simulink model "Sim4_CTM_Uncertainty_Controller"  (R2019b)
settings: Solver=ode45  StartTime=0.0  StopTime=10  MaxStep=0.001  RelTol=1e-3
StopFcn:
  | Colors=hsv(5)';
  | for i=1:5
  | plot(out.tout,out.R_UCTM(:,i),'color',Colors(:,i),'LineWidth',1.5)
  | hold on
  | end
  | grid on
  | legend('Joint1','Joint2','Joint3','Joint4','Joint5')
  | title(['Response Vs Input of Joints Via UCTM'])
  | xlabel('Time')
  | ylabel('Response')
  | 
  | 
  | 
  | %plot(out.tout,out.Results,'LineWidth',1.3)
  | %grid on
  | %legend('Joint1','Joint2','Joint3','Joint4','Joint5')
  | %xlabel('Response')
  | %ylabel('Time')
libraries: simulink x5
(part 1 of 3)
settings Model: Creator=baran  LastModifiedBy=baran

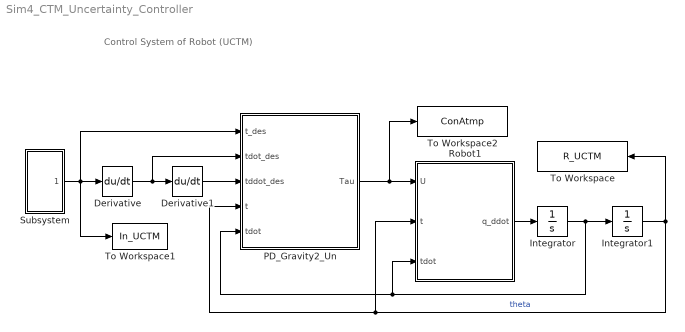
== system Sim4_CTM_Uncertainty_Controller ==
  note: Control System of Robot (UCTM)
  Derivative : Derivative
  Derivative1 : Derivative
  Integrator : Integrator  InitialCondition=[0 0 0 0 0]'
  Integrator1 : Integrator  InitialCondition=[-5 -4 -3 -2 -1]'
  PD_Gravity2_Un : MATLAB Function  TreatAsAtomicUnit=on
  Robot1 : MATLAB Function  TreatAsAtomicUnit=on
  Subsystem : Subsystem
  To Workspace : ToWorkspace  VariableName=R_UCTM  SampleTime=-1
  To Workspace1 : ToWorkspace  VariableName=In_UCTM  SampleTime=-1
  To Workspace2 : ToWorkspace  VariableName=ConAtmp  SampleTime=-1
  wires:
  PD_Gravity2_Un/1(Tau) -> To Workspace2/1, Robot1/1(U)
  Integrator/1 -> PD_Gravity2_Un/5(tdot), Robot1/3(tdot), Integrator1/1
  Robot1/1(q_ddot) -> Integrator/1
  Derivative/1 -> PD_Gravity2_Un/2(tdot_des), Derivative1/1
  Derivative1/1 -> PD_Gravity2_Un/3(tddot_des)
  Integrator1/1 -> PD_Gravity2_Un/4(t), Robot1/2(t), To Workspace/1  "theta"
  Subsystem/1(INPUT) -> PD_Gravity2_Un/1(t_des), To Workspace1/1, Derivative/1

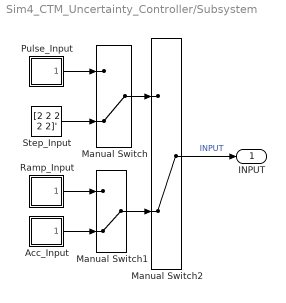
== system Sim4_CTM_Uncertainty_Controller/Subsystem ==
  Acc_Input : Subsystem
  Manual Switch : ManualSwitch  CurrentSetting=0
  Manual Switch1 : ManualSwitch  CurrentSetting=0
  Manual Switch2 : ManualSwitch  CurrentSetting=0
  Pulse_Input : Subsystem
  Ramp_Input : Subsystem
  Step_Input : Constant  Value=[2 2 2 2 2]'
  INPUT : Outport
  wires:
  Acc_Input/1(INPUT) -> Manual Switch1/2
  Ramp_Input/1(INPUT) -> Manual Switch1/1
  Pulse_Input/1(INPUT) -> Manual Switch/1
  Manual Switch2/1 -> INPUT/1  "INPUT"
  Manual Switch/1 -> Manual Switch2/1
  Manual Switch1/1 -> Manual Switch2/2
  Step_Input/1 -> Manual Switch/2

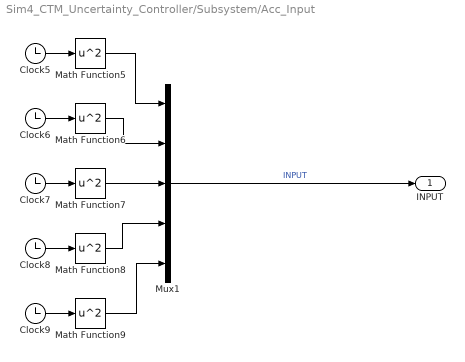
== system Sim4_CTM_Uncertainty_Controller/Subsystem/Acc_Input ==
  Clock{5..9} (5 alike) : Clock
  Math Function{5..9} (5 alike) : Math  Operator=square  SignedPower=off  SaturateOnIntegerOverflow=on
  Mux1 : Mux  Inputs=5
  INPUT : Outport
  wires:
  Math Function8/1 -> Mux1/4
  Math Function9/1 -> Mux1/5
  Clock5/1 -> Math Function5/1
  Math Function7/1 -> Mux1/3
  Clock9/1 -> Math Function9/1
  Math Function6/1 -> Mux1/2
  Clock8/1 -> Math Function8/1
  Clock7/1 -> Math Function7/1
  Math Function5/1 -> Mux1/1
  Clock6/1 -> Math Function6/1
  Mux1/1 -> INPUT/1  "INPUT"

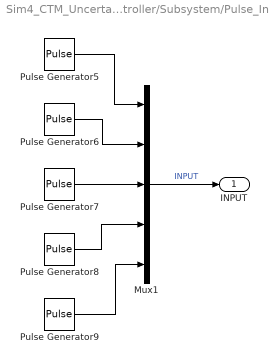
== system Sim4_CTM_Uncertainty_Controller/Subsystem/Pulse_Input ==
  Mux1 : Mux  Inputs=5
  Pulse Generator5 : DiscretePulseGenerator  PulseType=Time based  Period=10  PulseWidth=0.1
  Pulse Generator6 : DiscretePulseGenerator  PulseType=Time based  Amplitude=0.5  Period=10  PulseWidth=0.1
  Pulse Generator7 : DiscretePulseGenerator  PulseType=Time based  Amplitude=0.25  Period=10  PulseWidth=0.1
  Pulse Generator8 : DiscretePulseGenerator  PulseType=Time based  Amplitude=0.1  Period=10  PulseWidth=0.1
  Pulse Generator9 : DiscretePulseGenerator  PulseType=Time based  Amplitude=0.7  Period=10  PulseWidth=0.1
  INPUT : Outport
  wires:
  Pulse Generator7/1 -> Mux1/3
  Mux1/1 -> INPUT/1  "INPUT"
  Pulse Generator6/1 -> Mux1/2
  Pulse Generator5/1 -> Mux1/1
  Pulse Generator9/1 -> Mux1/5
  Pulse Generator8/1 -> Mux1/4

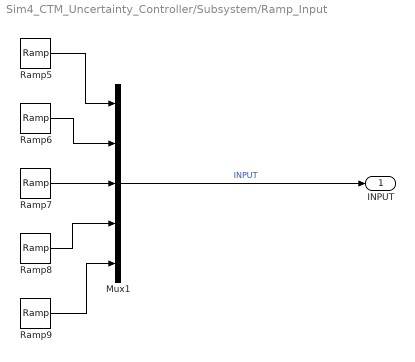
== system Sim4_CTM_Uncertainty_Controller/Subsystem/Ramp_Input ==
  Mux1 : Mux  Inputs=5
  Ramp{5..9} (5 alike) : simulink/Sources/Ramp  slope=2  start=0.0001  InitialOutput=0
  INPUT : Outport
  wires:
  Ramp5/1 -> Mux1/1
  Ramp6/1 -> Mux1/2
  Ramp8/1 -> Mux1/4
  Ramp7/1 -> Mux1/3
  Ramp9/1 -> Mux1/5
  Mux1/1 -> INPUT/1  "INPUT"
